simulink model "c00003M_harness"  (R2018a)
settings: Solver=ode3  StartTime=0.0  StopTime=10.0  RelTol=1e-3  EnableMultiTasking=on
undefined symbols (not defined in the file): b, DiscIntNeverNeededParam, J, K, L, PosMinimaW3, PosMinimaW4, R, sigbuilder_block
(part 59 of 73)

== stateflow chart c00003M_harness/M023/Cyber/WL1/Chart1 ==
  state Bajand_hasta_abajo
    entry: W = -1;
  state Bajando
    entry: W = -1;
  state Idle
    entry:W = 0;
  state Subiendo_hasta_arriba
    entry: W = 1;
  state Subiendo
    entry: W = 1;
  Subiendo -> Bajand_hasta_abajo [order 4] : [UI==4]
  Bajand_hasta_abajo -> Bajando [order 2] : [UI==3]
  Subiendo -> Bajando [order 3] : [UI==3]
  Bajando -> Bajand_hasta_abajo [order 2] : [UI==4]
  Idle -> Bajando [order 3] : [UI==3&&S>0]
  Subiendo_hasta_arriba -> Bajand_hasta_abajo [order 3] : [UI==4]
  Idle -> Bajand_hasta_abajo [order 4] : [UI==4&&S>0]
  Bajando -> Subiendo [order 3] : [UI==1]
  Subiendo_hasta_arriba -> Bajando [order 4] : [UI==3]
  Bajand_hasta_abajo -> Subiendo [order 4] : [UI==1]
  Bajand_hasta_abajo -> Idle [order 1] : [S<=0]
  Bajand_hasta_abajo -> Subiendo_hasta_arriba [order 3] : [UI==2]
  Bajando -> Idle [order 1] : [S<=0||UI==0]
  Bajando -> Subiendo_hasta_arriba [order 4] : [UI==2]
  (default) -> Idle
  Idle -> Subiendo_hasta_arriba [order 2] : [UI==2&&S<5]
  Idle -> Subiendo [order 1] : [UI == 1&&S<5]
  Subiendo -> Idle [order 1] : [S>=5||UI==0]
  Subiendo_hasta_arriba -> Idle [order 1] : [S >=5]
  Subiendo_hasta_arriba -> Subiendo [order 2] : [UI ==1]
  Subiendo -> Subiendo_hasta_arriba [order 2] : [UI==2]
  data: S input; UI input; W output double

== stateflow chart c00003M_harness/M023/Cyber/WL2/Chart1 ==
  state Bajand_hasta_abajo
    entry: W = -1;
  state Bajando
    entry: W = -1;
  state Idle
    entry:W = 0;
  state Subiendo_hasta_arriba
    entry: W = 1;
  state Subiendo
    entry: W = 1;
  Subiendo -> Bajand_hasta_abajo [order 4] : [UI==4]
  Bajand_hasta_abajo -> Bajando [order 2] : [UI==3]
  Subiendo -> Bajando [order 3] : [UI==3]
  Bajando -> Bajand_hasta_abajo [order 2] : [UI==4]
  Idle -> Bajando [order 3] : [UI==3&&S>PosMinW3]
  Subiendo_hasta_arriba -> Bajand_hasta_abajo [order 3] : [UI==4]
  Idle -> Bajand_hasta_abajo [order 4] : [UI==4&&S>PosMinW3]
  Bajando -> Subiendo [order 3] : [UI==1]
  Subiendo_hasta_arriba -> Bajando [order 4] : [UI==3]
  Bajand_hasta_abajo -> Subiendo [order 4] : [UI==1]
  Bajand_hasta_abajo -> Idle [order 1] : [S<=PosMinW3]
  Bajand_hasta_abajo -> Subiendo_hasta_arriba [order 3] : [UI==2]
  Bajando -> Idle [order 1] : [S<=PosMinW3||UI==0]
  Bajando -> Subiendo_hasta_arriba [order 4] : [UI==2]
  (default) -> Idle
  Idle -> Subiendo_hasta_arriba [order 2] : [UI==2&&S<5]
  Idle -> Subiendo [order 1] : [UI == 1&&S<5]
  Subiendo -> Idle [order 1] : [S>=5||UI==0]
  Subiendo_hasta_arriba -> Idle [order 1] : [S >=5]
  Subiendo_hasta_arriba -> Subiendo [order 2] : [UI ==1]
  Subiendo -> Subiendo_hasta_arriba [order 2] : [UI==2]
  data: S input; UI input; W output double; PosMinW3 input

== stateflow chart c00003M_harness/M023/Cyber/WL3/Chart2 ==
  state Bajand_hasta_abajo
    entry: W = -1;
  state Bajando
    entry: W = -1;
  state Idle
    entry:W = 0;
  state Subiendo_hasta_arriba
    entry: W = 1;
  state Subiendo
    entry: W = 1;
  Subiendo -> Bajand_hasta_abajo [order 4] : [UI==4]
  Bajand_hasta_abajo -> Bajando [order 2] : [UI==3]
  Subiendo -> Bajando [order 3] : [UI==3]
  Bajando -> Bajand_hasta_abajo [order 2] : [UI==4]
  Idle -> Bajando [order 3] : [UI==3&&S>PosMinW4]
  Subiendo_hasta_arriba -> Bajand_hasta_abajo [order 3] : [UI==4]
  Idle -> Bajand_hasta_abajo [order 4] : [UI==4&&S>PosMinW4]
  Bajando -> Subiendo [order 3] : [UI==1]
  Subiendo_hasta_arriba -> Bajando [order 4] : [UI==3]
  Bajand_hasta_abajo -> Subiendo [order 4] : [UI==1]
  Bajand_hasta_abajo -> Idle [order 1] : [S<=PosMinW4]
  Bajand_hasta_abajo -> Subiendo_hasta_arriba [order 3] : [UI==2]
  Bajando -> Idle [order 1] : [S<=PosMinW4||UI==0]
  Bajando -> Subiendo_hasta_arriba [order 4] : [UI==2]
  (default) -> Idle
  Idle -> Subiendo_hasta_arriba [order 2] : [UI==2&&S<5]
  Idle -> Subiendo [order 1] : [UI == 1&&S<5]
  Subiendo -> Idle [order 1] : [S>=5||UI==0]
  Subiendo_hasta_arriba -> Idle [order 1] : [S >=5]
  Subiendo_hasta_arriba -> Subiendo [order 2] : [UI ==1]
  Subiendo -> Subiendo_hasta_arriba [order 2] : [UI==2]
  data: S input; UI input; W output double; PosMinW4 input

== stateflow chart c00003M_harness/M024/Cyber/WL/Chart ==
  state Bajand_hasta_abajo
    entry: W = -1;
  state Bajando
    entry: W = -1;
  state Idle
    entry:W = 0;
  state Subiendo_hasta_arriba
    entry: W = 1;
  state Subiendo
    entry: W = 1;
  Subiendo -> Bajand_hasta_abajo [order 4] : [UI==4]
  Bajand_hasta_abajo -> Bajando [order 2] : [UI==3]
  Subiendo -> Bajando [order 3] : [UI==3]
  Bajando -> Bajand_hasta_abajo [order 2] : [UI==4]
  Idle -> Bajando [order 3] : [UI==3&&S>0]
  Subiendo_hasta_arriba -> Bajand_hasta_abajo [order 3] : [UI==4]
  Idle -> Bajand_hasta_abajo [order 4] : [UI==4&&S>0]
  Bajando -> Subiendo [order 3] : [UI==1]
  Subiendo_hasta_arriba -> Bajando [order 4] : [UI==3]
  Bajand_hasta_abajo -> Subiendo [order 4] : [UI==1]
  Bajand_hasta_abajo -> Idle [order 1] : [S<=0]
  Bajand_hasta_abajo -> Subiendo_hasta_arriba [order 3] : [UI==2]
  Bajando -> Idle [order 1] : [S<=0||UI==0]
  Bajando -> Subiendo_hasta_arriba [order 4] : [UI==2]
  (default) -> Idle
  Idle -> Subiendo_hasta_arriba [order 2] : [UI==2&&S<5]
  Idle -> Subiendo [order 1] : [UI == 1&&S<5]
  Subiendo -> Idle [order 1] : [S>=5||UI==0]
  Subiendo_hasta_arriba -> Idle [order 1] : [S >=5]
  Subiendo_hasta_arriba -> Subiendo [order 2] : [UI ==1]
  Subiendo -> Subiendo_hasta_arriba [order 2] : [UI==2]
  data: S input; UI input; W output double

== stateflow chart c00003M_harness/M024/Cyber/WL1/Chart1 ==
  state Bajand_hasta_abajo
    entry: W = -1;
  state Bajando
    entry: W = -1;
  state Idle
    entry:W = 1;
  state Subiendo_hasta_arriba
    entry: W = 1;
  state Subiendo
    entry: W = 1;
  Subiendo -> Bajand_hasta_abajo [order 4] : [UI==4]
  Bajand_hasta_abajo -> Bajando [order 2] : [UI==3]
  Subiendo -> Bajando [order 3] : [UI==3]
  Bajando -> Bajand_hasta_abajo [order 2] : [UI==4]
  Idle -> Bajando [order 3] : [UI==3&&S>0]
  Subiendo_hasta_arriba -> Bajand_hasta_abajo [order 3] : [UI==4]
  Idle -> Bajand_hasta_abajo [order 4] : [UI==4&&S>0]
  Bajando -> Subiendo [order 3] : [UI==1]
  Subiendo_hasta_arriba -> Bajando [order 4] : [UI==3]
  Bajand_hasta_abajo -> Subiendo [order 4] : [UI==1]
  Bajand_hasta_abajo -> Idle [order 1] : [S<=0]
  Bajand_hasta_abajo -> Subiendo_hasta_arriba [order 3] : [UI==2]
  Bajando -> Idle [order 1] : [S<=0||UI==0]
  Bajando -> Subiendo_hasta_arriba [order 4] : [UI==2]
  (default) -> Idle
  Idle -> Subiendo_hasta_arriba [order 2] : [UI==2&&S<5]
  Idle -> Subiendo [order 1] : [UI == 1&&S<5]
  Subiendo -> Idle [order 1] : [S>=5||UI==0]
  Subiendo_hasta_arriba -> Idle [order 1] : [S >=5]
  Subiendo_hasta_arriba -> Subiendo [order 2] : [UI ==1]
  Subiendo -> Subiendo_hasta_arriba [order 2] : [UI==2]
  data: S input; UI input; W output double

== stateflow chart c00003M_harness/M024/Cyber/WL2/Chart1 ==
  state Bajand_hasta_abajo
    entry: W = -1;
  state Bajando
    entry: W = -1;
  state Idle
    entry:W = 0;
  state Subiendo_hasta_arriba
    entry: W = 1;
  state Subiendo
    entry: W = 1;
  Subiendo -> Bajand_hasta_abajo [order 4] : [UI==4]
  Bajand_hasta_abajo -> Bajando [order 2] : [UI==3]
  Subiendo -> Bajando [order 3] : [UI==3]
  Bajando -> Bajand_hasta_abajo [order 2] : [UI==4]
  Idle -> Bajando [order 3] : [UI==3&&S>PosMinW3]
  Subiendo_hasta_arriba -> Bajand_hasta_abajo [order 3] : [UI==4]
  Idle -> Bajand_hasta_abajo [order 4] : [UI==4&&S>PosMinW3]
  Bajando -> Subiendo [order 3] : [UI==1]
  Subiendo_hasta_arriba -> Bajando [order 4] : [UI==3]
  Bajand_hasta_abajo -> Subiendo [order 4] : [UI==1]
  Bajand_hasta_abajo -> Idle [order 1] : [S<=PosMinW3]
  Bajand_hasta_abajo -> Subiendo_hasta_arriba [order 3] : [UI==2]
  Bajando -> Idle [order 1] : [S<=PosMinW3||UI==0]
  Bajando -> Subiendo_hasta_arriba [order 4] : [UI==2]
  (default) -> Idle
  Idle -> Subiendo_hasta_arriba [order 2] : [UI==2&&S<5]
  Idle -> Subiendo [order 1] : [UI == 1&&S<5]
  Subiendo -> Idle [order 1] : [S>=5||UI==0]
  Subiendo_hasta_arriba -> Idle [order 1] : [S >=5]
  Subiendo_hasta_arriba -> Subiendo [order 2] : [UI ==1]
  Subiendo -> Subiendo_hasta_arriba [order 2] : [UI==2]
  data: S input; UI input; W output double; PosMinW3 input

== stateflow chart c00003M_harness/M024/Cyber/WL3/Chart2 ==
  state Bajand_hasta_abajo
    entry: W = -1;
  state Bajando
    entry: W = -1;
  state Idle
    entry:W = 0;
  state Subiendo_hasta_arriba
    entry: W = 1;
  state Subiendo
    entry: W = 1;
  Subiendo -> Bajand_hasta_abajo [order 4] : [UI==4]
  Bajand_hasta_abajo -> Bajando [order 2] : [UI==3]
  Subiendo -> Bajando [order 3] : [UI==3]
  Bajando -> Bajand_hasta_abajo [order 2] : [UI==4]
  Idle -> Bajando [order 3] : [UI==3&&S>PosMinW4]
  Subiendo_hasta_arriba -> Bajand_hasta_abajo [order 3] : [UI==4]
  Idle -> Bajand_hasta_abajo [order 4] : [UI==4&&S>PosMinW4]
  Bajando -> Subiendo [order 3] : [UI==1]
  Subiendo_hasta_arriba -> Bajando [order 4] : [UI==3]
  Bajand_hasta_abajo -> Subiendo [order 4] : [UI==1]
  Bajand_hasta_abajo -> Idle [order 1] : [S<=PosMinW4]
  Bajand_hasta_abajo -> Subiendo_hasta_arriba [order 3] : [UI==2]
  Bajando -> Idle [order 1] : [S<=PosMinW4||UI==0]
  Bajando -> Subiendo_hasta_arriba [order 4] : [UI==2]
  (default) -> Idle
  Idle -> Subiendo_hasta_arriba [order 2] : [UI==2&&S<5]
  Idle -> Subiendo [order 1] : [UI == 1&&S<5]
  Subiendo -> Idle [order 1] : [S>=5||UI==0]
  Subiendo_hasta_arriba -> Idle [order 1] : [S >=5]
  Subiendo_hasta_arriba -> Subiendo [order 2] : [UI ==1]
  Subiendo -> Subiendo_hasta_arriba [order 2] : [UI==2]
  data: S input; UI input; W output double; PosMinW4 input

== stateflow chart c00003M_harness/M025/Cyber/WL/Chart ==
  state Bajand_hasta_abajo
    entry: W = -1;
  state Bajando
    entry: W = -1;
  state Idle
    entry:W = 0;
  state Subiendo_hasta_arriba
    entry: W = 1;
  state Subiendo
    entry: W = 1;
  Subiendo -> Bajand_hasta_abajo [order 4] : [UI==4]
  Bajand_hasta_abajo -> Bajando [order 2] : [UI==3]
  Subiendo -> Bajando [order 3] : [UI==3]
  Bajando -> Bajand_hasta_abajo [order 2] : [UI==4]
  Idle -> Bajando [order 3] : [UI==3&&S>0]
  Subiendo_hasta_arriba -> Bajand_hasta_abajo [order 3] : [UI==4]
  Idle -> Bajand_hasta_abajo [order 4] : [UI==4&&S>0]
  Bajando -> Subiendo [order 3] : [UI==1]
  Subiendo_hasta_arriba -> Bajando [order 4] : [UI==3]
  Bajand_hasta_abajo -> Subiendo [order 4] : [UI==1]
  Bajand_hasta_abajo -> Idle [order 1] : [S<=0]
  Bajand_hasta_abajo -> Subiendo_hasta_arriba [order 3] : [UI==2]
  Bajando -> Idle [order 1] : [S<=0||UI==0]
  Bajando -> Subiendo_hasta_arriba [order 4] : [UI==2]
  (default) -> Idle
  Idle -> Subiendo_hasta_arriba [order 2] : [UI==2&&S<5]
  Idle -> Subiendo [order 1] : [UI == 1&&S<5]
  Subiendo -> Idle [order 1] : [S>=5||UI==0]
  Subiendo_hasta_arriba -> Idle [order 1] : [S >=5]
  Subiendo_hasta_arriba -> Subiendo [order 2] : [UI ==1]
  Subiendo -> Subiendo_hasta_arriba [order 2] : [UI==2]
  data: S input; UI input; W output double

== stateflow chart c00003M_harness/M025/Cyber/WL1/Chart1 ==
  state Bajand_hasta_abajo
    entry: W = -1;
  state Bajando
    entry: W = -1;
  state Idle
    entry:W = 0;
  state Subiendo_hasta_arriba
    entry: W = 1;
  state Subiendo
    entry: W = 1;
  Subiendo -> Bajand_hasta_abajo [order 4] : [UI==4]
  Bajand_hasta_abajo -> Bajando [order 2] : [UI==3]
  Subiendo -> Bajando [order 3] : [UI==3]
  Bajando -> Bajand_hasta_abajo [order 2] : [UI==4]
  Idle -> Bajando [order 3] : [UI==3&&S>0]
  Subiendo_hasta_arriba -> Bajand_hasta_abajo [order 3] : [UI==4]
  Idle -> Bajand_hasta_abajo [order 4] : [UI==4&&S>0]
  Bajando -> Subiendo [order 3] : [UI==1]
  Subiendo_hasta_arriba -> Bajando [order 4] : [UI==3]
  Bajand_hasta_abajo -> Subiendo [order 4] : [UI==1]
  Bajand_hasta_abajo -> Idle [order 1] : [S<=0]
  Bajand_hasta_abajo -> Subiendo_hasta_arriba [order 3] : [UI==2]
  Bajando -> Idle [order 1] : [S<=0||UI==0]
  Bajando -> Subiendo_hasta_arriba [order 4] : [UI==2]
  (default) -> Idle
  Idle -> Subiendo_hasta_arriba [order 2] : [UI==2&&S<5]
  Idle -> Subiendo [order 1] : [UI == 1&&S<5]
  Subiendo -> Idle [order 1] : [S>=5||UI==0]
  Subiendo_hasta_arriba -> Idle [order 1] : [S >=5]
  Subiendo_hasta_arriba -> Subiendo [order 2] : [UI ==1]
  Subiendo -> Subiendo_hasta_arriba [order 2] : [UI==2]
  data: S input; UI input; W output double

== stateflow chart c00003M_harness/M025/Cyber/WL2/Chart1 ==
  state Bajand_hasta_abajo
    entry: W = -1;
  state Bajando
    entry: W = -1;
  state Idle
    entry:W = 1;
  state Subiendo_hasta_arriba
    entry: W = 1;
  state Subiendo
    entry: W = 1;
  Subiendo -> Bajand_hasta_abajo [order 4] : [UI==4]
  Bajand_hasta_abajo -> Bajando [order 2] : [UI==3]
  Subiendo -> Bajando [order 3] : [UI==3]
  Bajando -> Bajand_hasta_abajo [order 2] : [UI==4]
  Idle -> Bajando [order 3] : [UI==3&&S>PosMinW3]
  Subiendo_hasta_arriba -> Bajand_hasta_abajo [order 3] : [UI==4]
  Idle -> Bajand_hasta_abajo [order 4] : [UI==4&&S>PosMinW3]
  Bajando -> Subiendo [order 3] : [UI==1]
  Subiendo_hasta_arriba -> Bajando [order 4] : [UI==3]
  Bajand_hasta_abajo -> Subiendo [order 4] : [UI==1]
  Bajand_hasta_abajo -> Idle [order 1] : [S<=PosMinW3]
  Bajand_hasta_abajo -> Subiendo_hasta_arriba [order 3] : [UI==2]
  Bajando -> Idle [order 1] : [S<=PosMinW3||UI==0]
  Bajando -> Subiendo_hasta_arriba [order 4] : [UI==2]
  (default) -> Idle
  Idle -> Subiendo_hasta_arriba [order 2] : [UI==2&&S<5]
  Idle -> Subiendo [order 1] : [UI == 1&&S<5]
  Subiendo -> Idle [order 1] : [S>=5||UI==0]
  Subiendo_hasta_arriba -> Idle [order 1] : [S >=5]
  Subiendo_hasta_arriba -> Subiendo [order 2] : [UI ==1]
  Subiendo -> Subiendo_hasta_arriba [order 2] : [UI==2]
  data: S input; UI input; W output double; PosMinW3 input

== stateflow chart c00003M_harness/M025/Cyber/WL3/Chart2 ==
  state Bajand_hasta_abajo
    entry: W = -1;
  state Bajando
    entry: W = -1;
  state Idle
    entry:W = 0;
  state Subiendo_hasta_arriba
    entry: W = 1;
  state Subiendo
    entry: W = 1;
  Subiendo -> Bajand_hasta_abajo [order 4] : [UI==4]
  Bajand_hasta_abajo -> Bajando [order 2] : [UI==3]
  Subiendo -> Bajando [order 3] : [UI==3]
  Bajando -> Bajand_hasta_abajo [order 2] : [UI==4]
  Idle -> Bajando [order 3] : [UI==3&&S>PosMinW4]
  Subiendo_hasta_arriba -> Bajand_hasta_abajo [order 3] : [UI==4]
  Idle -> Bajand_hasta_abajo [order 4] : [UI==4&&S>PosMinW4]
  Bajando -> Subiendo [order 3] : [UI==1]
  Subiendo_hasta_arriba -> Bajando [order 4] : [UI==3]
  Bajand_hasta_abajo -> Subiendo [order 4] : [UI==1]
  Bajand_hasta_abajo -> Idle [order 1] : [S<=PosMinW4]
  Bajand_hasta_abajo -> Subiendo_hasta_arriba [order 3] : [UI==2]
  Bajando -> Idle [order 1] : [S<=PosMinW4||UI==0]
  Bajando -> Subiendo_hasta_arriba [order 4] : [UI==2]
  (default) -> Idle
  Idle -> Subiendo_hasta_arriba [order 2] : [UI==2&&S<5]
  Idle -> Subiendo [order 1] : [UI == 1&&S<5]
  Subiendo -> Idle [order 1] : [S>=5||UI==0]
  Subiendo_hasta_arriba -> Idle [order 1] : [S >=5]
  Subiendo_hasta_arriba -> Subiendo [order 2] : [UI ==1]
  Subiendo -> Subiendo_hasta_arriba [order 2] : [UI==2]
  data: S input; UI input; W output double; PosMinW4 input

== stateflow chart c00003M_harness/M026/Cyber/WL/Chart ==
  state Bajand_hasta_abajo
    entry: W = -1;
  state Bajando
    entry: W = -1;
  state Idle
    entry:W = 0;
  state Subiendo_hasta_arriba
    entry: W = 1;
  state Subiendo
    entry: W = 1;
  Subiendo -> Bajand_hasta_abajo [order 4] : [UI==4]
  Bajand_hasta_abajo -> Bajando [order 2] : [UI==3]
  Subiendo -> Bajando [order 3] : [UI==3]
  Bajando -> Bajand_hasta_abajo [order 2] : [UI==4]
  Idle -> Bajando [order 3] : [UI==3&&S>0]
  Subiendo_hasta_arriba -> Bajand_hasta_abajo [order 3] : [UI==4]
  Idle -> Bajand_hasta_abajo [order 4] : [UI==4&&S>0]
  Bajando -> Subiendo [order 3] : [UI==1]
  Subiendo_hasta_arriba -> Bajando [order 4] : [UI==3]
  Bajand_hasta_abajo -> Subiendo [order 4] : [UI==1]
  Bajand_hasta_abajo -> Idle [order 1] : [S<=0]
  Bajand_hasta_abajo -> Subiendo_hasta_arriba [order 3] : [UI==2]
  Bajando -> Idle [order 1] : [S<=0||UI==0]
  Bajando -> Subiendo_hasta_arriba [order 4] : [UI==2]
  (default) -> Idle
  Idle -> Subiendo_hasta_arriba [order 2] : [UI==2&&S<5]
  Idle -> Subiendo [order 1] : [UI == 1&&S<5]
  Subiendo -> Idle [order 1] : [S>=5||UI==0]
  Subiendo_hasta_arriba -> Idle [order 1] : [S >=5]
  Subiendo_hasta_arriba -> Subiendo [order 2] : [UI ==1]
  Subiendo -> Subiendo_hasta_arriba [order 2] : [UI==2]
  data: S input; UI input; W output double

== stateflow chart c00003M_harness/M026/Cyber/WL1/Chart1 ==
  state Bajand_hasta_abajo
    entry: W = -1;
  state Bajando
    entry: W = -1;
  state Idle
    entry:W = 0;
  state Subiendo_hasta_arriba
    entry: W = 1;
  state Subiendo
    entry: W = 1;
  Subiendo -> Bajand_hasta_abajo [order 4] : [UI==4]
  Bajand_hasta_abajo -> Bajando [order 2] : [UI==3]
  Subiendo -> Bajando [order 3] : [UI==3]
  Bajando -> Bajand_hasta_abajo [order 2] : [UI==4]
  Idle -> Bajando [order 3] : [UI==3&&S>0]
  Subiendo_hasta_arriba -> Bajand_hasta_abajo [order 3] : [UI==4]
  Idle -> Bajand_hasta_abajo [order 4] : [UI==4&&S>0]
  Bajando -> Subiendo [order 3] : [UI==1]
  Subiendo_hasta_arriba -> Bajando [order 4] : [UI==3]
  Bajand_hasta_abajo -> Subiendo [order 4] : [UI==1]
  Bajand_hasta_abajo -> Idle [order 1] : [S<=0]
  Bajand_hasta_abajo -> Subiendo_hasta_arriba [order 3] : [UI==2]
  Bajando -> Idle [order 1] : [S<=0||UI==0]
  Bajando -> Subiendo_hasta_arriba [order 4] : [UI==2]
  (default) -> Idle
  Idle -> Subiendo_hasta_arriba [order 2] : [UI==2&&S<5]
  Idle -> Subiendo [order 1] : [UI == 1&&S<5]
  Subiendo -> Idle [order 1] : [S>=5||UI==0]
  Subiendo_hasta_arriba -> Idle [order 1] : [S >=5]
  Subiendo_hasta_arriba -> Subiendo [order 2] : [UI ==1]
  Subiendo -> Subiendo_hasta_arriba [order 2] : [UI==2]
  data: S input; UI input; W output double

== stateflow chart c00003M_harness/M026/Cyber/WL2/Chart1 ==
  state Bajand_hasta_abajo
    entry: W = -1;
  state Bajando
    entry: W = -1;
  state Idle
    entry:W = 0;
  state Subiendo_hasta_arriba
    entry: W = 1;
  state Subiendo
    entry: W = 1;
  Subiendo -> Bajand_hasta_abajo [order 4] : [UI==4]
  Bajand_hasta_abajo -> Bajando [order 2] : [UI==3]
  Subiendo -> Bajando [order 3] : [UI==3]
  Bajando -> Bajand_hasta_abajo [order 2] : [UI==4]
  Idle -> Bajando [order 3] : [UI==3&&S>PosMinW3]
  Subiendo_hasta_arriba -> Bajand_hasta_abajo [order 3] : [UI==4]
  Idle -> Bajand_hasta_abajo [order 4] : [UI==4&&S>PosMinW3]
  Bajando -> Subiendo [order 3] : [UI==1]
  Subiendo_hasta_arriba -> Bajando [order 4] : [UI==3]
  Bajand_hasta_abajo -> Subiendo [order 4] : [UI==1]
  Bajand_hasta_abajo -> Idle [order 1] : [S<=PosMinW3]
  Bajand_hasta_abajo -> Subiendo_hasta_arriba [order 3] : [UI==2]
  Bajando -> Idle [order 1] : [S<=PosMinW3||UI==0]
  Bajando -> Subiendo_hasta_arriba [order 4] : [UI==2]
  (default) -> Idle
  Idle -> Subiendo_hasta_arriba [order 2] : [UI==2&&S<5]
  Idle -> Subiendo [order 1] : [UI == 1&&S<5]
  Subiendo -> Idle [order 1] : [S>=5||UI==0]
  Subiendo_hasta_arriba -> Idle [order 1] : [S >=5]
  Subiendo_hasta_arriba -> Subiendo [order 2] : [UI ==1]
  Subiendo -> Subiendo_hasta_arriba [order 2] : [UI==2]
  data: S input; UI input; W output double; PosMinW3 input

== stateflow chart c00003M_harness/M026/Cyber/WL3/Chart2 ==
  state Bajand_hasta_abajo
    entry: W = -1;
  state Bajando
    entry: W = -1;
  state Idle
    entry:W = 1;
  state Subiendo_hasta_arriba
    entry: W = 1;
  state Subiendo
    entry: W = 1;
  Subiendo -> Bajand_hasta_abajo [order 4] : [UI==4]
  Bajand_hasta_abajo -> Bajando [order 2] : [UI==3]
  Subiendo -> Bajando [order 3] : [UI==3]
  Bajando -> Bajand_hasta_abajo [order 2] : [UI==4]
  Idle -> Bajando [order 3] : [UI==3&&S>PosMinW4]
  Subiendo_hasta_arriba -> Bajand_hasta_abajo [order 3] : [UI==4]
  Idle -> Bajand_hasta_abajo [order 4] : [UI==4&&S>PosMinW4]
  Bajando -> Subiendo [order 3] : [UI==1]
  Subiendo_hasta_arriba -> Bajando [order 4] : [UI==3]
  Bajand_hasta_abajo -> Subiendo [order 4] : [UI==1]
  Bajand_hasta_abajo -> Idle [order 1] : [S<=PosMinW4]
  Bajand_hasta_abajo -> Subiendo_hasta_arriba [order 3] : [UI==2]
  Bajando -> Idle [order 1] : [S<=PosMinW4||UI==0]
  Bajando -> Subiendo_hasta_arriba [order 4] : [UI==2]
  (default) -> Idle
  Idle -> Subiendo_hasta_arriba [order 2] : [UI==2&&S<5]
  Idle -> Subiendo [order 1] : [UI == 1&&S<5]
  Subiendo -> Idle [order 1] : [S>=5||UI==0]
  Subiendo_hasta_arriba -> Idle [order 1] : [S >=5]
  Subiendo_hasta_arriba -> Subiendo [order 2] : [UI ==1]
  Subiendo -> Subiendo_hasta_arriba [order 2] : [UI==2]
  data: S input; UI input; W output double; PosMinW4 input

== stateflow chart c00003M_harness/M027/Cyber/WL/Chart ==
  state Bajand_hasta_abajo
    entry: W = -1;
  state Bajando
    entry: W = -1;
  state Idle
    entry:W = 0;
  state Subiendo_hasta_arriba
    entry: W = 1;
  state Subiendo
    entry: W = 0;
  Subiendo -> Bajand_hasta_abajo [order 4] : [UI==4]
  Bajand_hasta_abajo -> Bajando [order 2] : [UI==3]
  Subiendo -> Bajando [order 3] : [UI==3]
  Bajando -> Bajand_hasta_abajo [order 2] : [UI==4]
  Idle -> Bajando [order 3] : [UI==3&&S>0]
  Subiendo_hasta_arriba -> Bajand_hasta_abajo [order 3] : [UI==4]
  Idle -> Bajand_hasta_abajo [order 4] : [UI==4&&S>0]
  Bajando -> Subiendo [order 3] : [UI==1]
  Subiendo_hasta_arriba -> Bajando [order 4] : [UI==3]
  Bajand_hasta_abajo -> Subiendo [order 4] : [UI==1]
  Bajand_hasta_abajo -> Idle [order 1] : [S<=0]
  Bajand_hasta_abajo -> Subiendo_hasta_arriba [order 3] : [UI==2]
  Bajando -> Idle [order 1] : [S<=0||UI==0]
  Bajando -> Subiendo_hasta_arriba [order 4] : [UI==2]
  (default) -> Idle
  Idle -> Subiendo_hasta_arriba [order 2] : [UI==2&&S<5]
  Idle -> Subiendo [order 1] : [UI == 1&&S<5]
  Subiendo -> Idle [order 1] : [S>=5||UI==0]
  Subiendo_hasta_arriba -> Idle [order 1] : [S >=5]
  Subiendo_hasta_arriba -> Subiendo [order 2] : [UI ==1]
  Subiendo -> Subiendo_hasta_arriba [order 2] : [UI==2]
  data: S input; UI input; W output double

== stateflow chart c00003M_harness/M027/Cyber/WL1/Chart1 ==
  state Bajand_hasta_abajo
    entry: W = -1;
  state Bajando
    entry: W = -1;
  state Idle
    entry:W = 0;
  state Subiendo_hasta_arriba
    entry: W = 1;
  state Subiendo
    entry: W = 1;
  Subiendo -> Bajand_hasta_abajo [order 4] : [UI==4]
  Bajand_hasta_abajo -> Bajando [order 2] : [UI==3]
  Subiendo -> Bajando [order 3] : [UI==3]
  Bajando -> Bajand_hasta_abajo [order 2] : [UI==4]
  Idle -> Bajando [order 3] : [UI==3&&S>0]
  Subiendo_hasta_arriba -> Bajand_hasta_abajo [order 3] : [UI==4]
  Idle -> Bajand_hasta_abajo [order 4] : [UI==4&&S>0]
  Bajando -> Subiendo [order 3] : [UI==1]
  Subiendo_hasta_arriba -> Bajando [order 4] : [UI==3]
  Bajand_hasta_abajo -> Subiendo [order 4] : [UI==1]
  Bajand_hasta_abajo -> Idle [order 1] : [S<=0]
  Bajand_hasta_abajo -> Subiendo_hasta_arriba [order 3] : [UI==2]
  Bajando -> Idle [order 1] : [S<=0||UI==0]
  Bajando -> Subiendo_hasta_arriba [order 4] : [UI==2]
  (default) -> Idle
  Idle -> Subiendo_hasta_arriba [order 2] : [UI==2&&S<5]
  Idle -> Subiendo [order 1] : [UI == 1&&S<5]
  Subiendo -> Idle [order 1] : [S>=5||UI==0]
  Subiendo_hasta_arriba -> Idle [order 1] : [S >=5]
  Subiendo_hasta_arriba -> Subiendo [order 2] : [UI ==1]
  Subiendo -> Subiendo_hasta_arriba [order 2] : [UI==2]
  data: S input; UI input; W output double

== stateflow chart c00003M_harness/M027/Cyber/WL2/Chart1 ==
  state Bajand_hasta_abajo
    entry: W = -1;
  state Bajando
    entry: W = -1;
  state Idle
    entry:W = 0;
  state Subiendo_hasta_arriba
    entry: W = 1;
  state Subiendo
    entry: W = 1;
  Subiendo -> Bajand_hasta_abajo [order 4] : [UI==4]
  Bajand_hasta_abajo -> Bajando [order 2] : [UI==3]
  Subiendo -> Bajando [order 3] : [UI==3]
  Bajando -> Bajand_hasta_abajo [order 2] : [UI==4]
  Idle -> Bajando [order 3] : [UI==3&&S>PosMinW3]
  Subiendo_hasta_arriba -> Bajand_hasta_abajo [order 3] : [UI==4]
  Idle -> Bajand_hasta_abajo [order 4] : [UI==4&&S>PosMinW3]
  Bajando -> Subiendo [order 3] : [UI==1]
  Subiendo_hasta_arriba -> Bajando [order 4] : [UI==3]
  Bajand_hasta_abajo -> Subiendo [order 4] : [UI==1]
  Bajand_hasta_abajo -> Idle [order 1] : [S<=PosMinW3]
  Bajand_hasta_abajo -> Subiendo_hasta_arriba [order 3] : [UI==2]
  Bajando -> Idle [order 1] : [S<=PosMinW3||UI==0]
  Bajando -> Subiendo_hasta_arriba [order 4] : [UI==2]
  (default) -> Idle
  Idle -> Subiendo_hasta_arriba [order 2] : [UI==2&&S<5]
  Idle -> Subiendo [order 1] : [UI == 1&&S<5]
  Subiendo -> Idle [order 1] : [S>=5||UI==0]
  Subiendo_hasta_arriba -> Idle [order 1] : [S >=5]
  Subiendo_hasta_arriba -> Subiendo [order 2] : [UI ==1]
  Subiendo -> Subiendo_hasta_arriba [order 2] : [UI==2]
  data: S input; UI input; W output double; PosMinW3 input

== stateflow chart c00003M_harness/M027/Cyber/WL3/Chart2 ==
  state Bajand_hasta_abajo
    entry: W = -1;
  state Bajando
    entry: W = -1;
  state Idle
    entry:W = 0;
  state Subiendo_hasta_arriba
    entry: W = 1;
  state Subiendo
    entry: W = 1;
  Subiendo -> Bajand_hasta_abajo [order 4] : [UI==4]
  Bajand_hasta_abajo -> Bajando [order 2] : [UI==3]
  Subiendo -> Bajando [order 3] : [UI==3]
  Bajando -> Bajand_hasta_abajo [order 2] : [UI==4]
  Idle -> Bajando [order 3] : [UI==3&&S>PosMinW4]
  Subiendo_hasta_arriba -> Bajand_hasta_abajo [order 3] : [UI==4]
  Idle -> Bajand_hasta_abajo [order 4] : [UI==4&&S>PosMinW4]
  Bajando -> Subiendo [order 3] : [UI==1]
  Subiendo_hasta_arriba -> Bajando [order 4] : [UI==3]
  Bajand_hasta_abajo -> Subiendo [order 4] : [UI==1]
  Bajand_hasta_abajo -> Idle [order 1] : [S<=PosMinW4]
  Bajand_hasta_abajo -> Subiendo_hasta_arriba [order 3] : [UI==2]
  Bajando -> Idle [order 1] : [S<=PosMinW4||UI==0]
  Bajando -> Subiendo_hasta_arriba [order 4] : [UI==2]
  (default) -> Idle
  Idle -> Subiendo_hasta_arriba [order 2] : [UI==2&&S<5]
  Idle -> Subiendo [order 1] : [UI == 1&&S<5]
  Subiendo -> Idle [order 1] : [S>=5||UI==0]
  Subiendo_hasta_arriba -> Idle [order 1] : [S >=5]
  Subiendo_hasta_arriba -> Subiendo [order 2] : [UI ==1]
  Subiendo -> Subiendo_hasta_arriba [order 2] : [UI==2]
  data: S input; UI input; W output double; PosMinW4 input

== stateflow chart c00003M_harness/M028/Cyber/WL/Chart ==
  state Bajand_hasta_abajo
    entry: W = -1;
  state Bajando
    entry: W = -1;
  state Idle
    entry:W = 0;
  state Subiendo_hasta_arriba
    entry: W = 1;
  state Subiendo
    entry: W = 1;
  Subiendo -> Bajand_hasta_abajo [order 4] : [UI==4]
  Bajand_hasta_abajo -> Bajando [order 2] : [UI==3]
  Subiendo -> Bajando [order 3] : [UI==3]
  Bajando -> Bajand_hasta_abajo [order 2] : [UI==4]
  Idle -> Bajando [order 3] : [UI==3&&S>0]
  Subiendo_hasta_arriba -> Bajand_hasta_abajo [order 3] : [UI==4]
  Idle -> Bajand_hasta_abajo [order 4] : [UI==4&&S>0]
  Bajando -> Subiendo [order 3] : [UI==1]
  Subiendo_hasta_arriba -> Bajando [order 4] : [UI==3]
  Bajand_hasta_abajo -> Subiendo [order 4] : [UI==1]
  Bajand_hasta_abajo -> Idle [order 1] : [S<=0]
  Bajand_hasta_abajo -> Subiendo_hasta_arriba [order 3] : [UI==2]
  Bajando -> Idle [order 1] : [S<=0||UI==0]
  Bajando -> Subiendo_hasta_arriba [order 4] : [UI==2]
  (default) -> Idle
  Idle -> Subiendo_hasta_arriba [order 2] : [UI==2&&S<5]
  Idle -> Subiendo [order 1] : [UI == 1&&S<5]
  Subiendo -> Idle [order 1] : [S>=5||UI==0]
  Subiendo_hasta_arriba -> Idle [order 1] : [S >=5]
  Subiendo_hasta_arriba -> Subiendo [order 2] : [UI ==1]
  Subiendo -> Subiendo_hasta_arriba [order 2] : [UI==2]
  data: S input; UI input; W output double

== stateflow chart c00003M_harness/M028/Cyber/WL1/Chart1 ==
  state Bajand_hasta_abajo
    entry: W = -1;
  state Bajando
    entry: W = -1;
  state Idle
    entry:W = 0;
  state Subiendo_hasta_arriba
    entry: W = 1;
  state Subiendo
    entry: W = 0;
  Subiendo -> Bajand_hasta_abajo [order 4] : [UI==4]
  Bajand_hasta_abajo -> Bajando [order 2] : [UI==3]
  Subiendo -> Bajando [order 3] : [UI==3]
  Bajando -> Bajand_hasta_abajo [order 2] : [UI==4]
  Idle -> Bajando [order 3] : [UI==3&&S>0]
  Subiendo_hasta_arriba -> Bajand_hasta_abajo [order 3] : [UI==4]
  Idle -> Bajand_hasta_abajo [order 4] : [UI==4&&S>0]
  Bajando -> Subiendo [order 3] : [UI==1]
  Subiendo_hasta_arriba -> Bajando [order 4] : [UI==3]
  Bajand_hasta_abajo -> Subiendo [order 4] : [UI==1]
  Bajand_hasta_abajo -> Idle [order 1] : [S<=0]
  Bajand_hasta_abajo -> Subiendo_hasta_arriba [order 3] : [UI==2]
  Bajando -> Idle [order 1] : [S<=0||UI==0]
  Bajando -> Subiendo_hasta_arriba [order 4] : [UI==2]
  (default) -> Idle
  Idle -> Subiendo_hasta_arriba [order 2] : [UI==2&&S<5]
  Idle -> Subiendo [order 1] : [UI == 1&&S<5]
  Subiendo -> Idle [order 1] : [S>=5||UI==0]
  Subiendo_hasta_arriba -> Idle [order 1] : [S >=5]
  Subiendo_hasta_arriba -> Subiendo [order 2] : [UI ==1]
  Subiendo -> Subiendo_hasta_arriba [order 2] : [UI==2]
  data: S input; UI input; W output double

== stateflow chart c00003M_harness/M028/Cyber/WL2/Chart1 ==
  state Bajand_hasta_abajo
    entry: W = -1;
  state Bajando
    entry: W = -1;
  state Idle
    entry:W = 0;
  state Subiendo_hasta_arriba
    entry: W = 1;
  state Subiendo
    entry: W = 1;
  Subiendo -> Bajand_hasta_abajo [order 4] : [UI==4]
  Bajand_hasta_abajo -> Bajando [order 2] : [UI==3]
  Subiendo -> Bajando [order 3] : [UI==3]
  Bajando -> Bajand_hasta_abajo [order 2] : [UI==4]
  Idle -> Bajando [order 3] : [UI==3&&S>PosMinW3]
  Subiendo_hasta_arriba -> Bajand_hasta_abajo [order 3] : [UI==4]
  Idle -> Bajand_hasta_abajo [order 4] : [UI==4&&S>PosMinW3]
  Bajando -> Subiendo [order 3] : [UI==1]
  Subiendo_hasta_arriba -> Bajando [order 4] : [UI==3]
  Bajand_hasta_abajo -> Subiendo [order 4] : [UI==1]
  Bajand_hasta_abajo -> Idle [order 1] : [S<=PosMinW3]
  Bajand_hasta_abajo -> Subiendo_hasta_arriba [order 3] : [UI==2]
  Bajando -> Idle [order 1] : [S<=PosMinW3||UI==0]
  Bajando -> Subiendo_hasta_arriba [order 4] : [UI==2]
  (default) -> Idle
  Idle -> Subiendo_hasta_arriba [order 2] : [UI==2&&S<5]
  Idle -> Subiendo [order 1] : [UI == 1&&S<5]
  Subiendo -> Idle [order 1] : [S>=5||UI==0]
  Subiendo_hasta_arriba -> Idle [order 1] : [S >=5]
  Subiendo_hasta_arriba -> Subiendo [order 2] : [UI ==1]
  Subiendo -> Subiendo_hasta_arriba [order 2] : [UI==2]
  data: S input; UI input; W output double; PosMinW3 input

== stateflow chart c00003M_harness/M028/Cyber/WL3/Chart2 ==
  state Bajand_hasta_abajo
    entry: W = -1;
  state Bajando
    entry: W = -1;
  state Idle
    entry:W = 0;
  state Subiendo_hasta_arriba
    entry: W = 1;
  state Subiendo
    entry: W = 1;
  Subiendo -> Bajand_hasta_abajo [order 4] : [UI==4]
  Bajand_hasta_abajo -> Bajando [order 2] : [UI==3]
  Subiendo -> Bajando [order 3] : [UI==3]
  Bajando -> Bajand_hasta_abajo [order 2] : [UI==4]
  Idle -> Bajando [order 3] : [UI==3&&S>PosMinW4]
  Subiendo_hasta_arriba -> Bajand_hasta_abajo [order 3] : [UI==4]
  Idle -> Bajand_hasta_abajo [order 4] : [UI==4&&S>PosMinW4]
  Bajando -> Subiendo [order 3] : [UI==1]
  Subiendo_hasta_arriba -> Bajando [order 4] : [UI==3]
  Bajand_hasta_abajo -> Subiendo [order 4] : [UI==1]
  Bajand_hasta_abajo -> Idle [order 1] : [S<=PosMinW4]
  Bajand_hasta_abajo -> Subiendo_hasta_arriba [order 3] : [UI==2]
  Bajando -> Idle [order 1] : [S<=PosMinW4||UI==0]
  Bajando -> Subiendo_hasta_arriba [order 4] : [UI==2]
  (default) -> Idle
  Idle -> Subiendo_hasta_arriba [order 2] : [UI==2&&S<5]
  Idle -> Subiendo [order 1] : [UI == 1&&S<5]
  Subiendo -> Idle [order 1] : [S>=5||UI==0]
  Subiendo_hasta_arriba -> Idle [order 1] : [S >=5]
  Subiendo_hasta_arriba -> Subiendo [order 2] : [UI ==1]
  Subiendo -> Subiendo_hasta_arriba [order 2] : [UI==2]
  data: S input; UI input; W output double; PosMinW4 input

== stateflow chart c00003M_harness/M029/Cyber/WL/Chart ==
  state Bajand_hasta_abajo
    entry: W = -1;
  state Bajando
    entry: W = -1;
  state Idle
    entry:W = 0;
  state Subiendo_hasta_arriba
    entry: W = 1;
  state Subiendo
    entry: W = 1;
  Subiendo -> Bajand_hasta_abajo [order 4] : [UI==4]
  Bajand_hasta_abajo -> Bajando [order 2] : [UI==3]
  Subiendo -> Bajando [order 3] : [UI==3]
  Bajando -> Bajand_hasta_abajo [order 2] : [UI==4]
  Idle -> Bajando [order 3] : [UI==3&&S>0]
  Subiendo_hasta_arriba -> Bajand_hasta_abajo [order 3] : [UI==4]
  Idle -> Bajand_hasta_abajo [order 4] : [UI==4&&S>0]
  Bajando -> Subiendo [order 3] : [UI==1]
  Subiendo_hasta_arriba -> Bajando [order 4] : [UI==3]
  Bajand_hasta_abajo -> Subiendo [order 4] : [UI==1]
  Bajand_hasta_abajo -> Idle [order 1] : [S<=0]
  Bajand_hasta_abajo -> Subiendo_hasta_arriba [order 3] : [UI==2]
  Bajando -> Idle [order 1] : [S<=0||UI==0]
  Bajando -> Subiendo_hasta_arriba [order 4] : [UI==2]
  (default) -> Idle
  Idle -> Subiendo_hasta_arriba [order 2] : [UI==2&&S<5]
  Idle -> Subiendo [order 1] : [UI == 1&&S<5]
  Subiendo -> Idle [order 1] : [S>=5||UI==0]
  Subiendo_hasta_arriba -> Idle [order 1] : [S >=5]
  Subiendo_hasta_arriba -> Subiendo [order 2] : [UI ==1]
  Subiendo -> Subiendo_hasta_arriba [order 2] : [UI==2]
  data: S input; UI input; W output double

== stateflow chart c00003M_harness/M029/Cyber/WL1/Chart1 ==
  state Bajand_hasta_abajo
    entry: W = -1;
  state Bajando
    entry: W = -1;
  state Idle
    entry:W = 0;
  state Subiendo_hasta_arriba
    entry: W = 1;
  state Subiendo
    entry: W = 1;
  Subiendo -> Bajand_hasta_abajo [order 4] : [UI==4]
  Bajand_hasta_abajo -> Bajando [order 2] : [UI==3]
  Subiendo -> Bajando [order 3] : [UI==3]
  Bajando -> Bajand_hasta_abajo [order 2] : [UI==4]
  Idle -> Bajando [order 3] : [UI==3&&S>0]
  Subiendo_hasta_arriba -> Bajand_hasta_abajo [order 3] : [UI==4]
  Idle -> Bajand_hasta_abajo [order 4] : [UI==4&&S>0]
  Bajando -> Subiendo [order 3] : [UI==1]
  Subiendo_hasta_arriba -> Bajando [order 4] : [UI==3]
  Bajand_hasta_abajo -> Subiendo [order 4] : [UI==1]
  Bajand_hasta_abajo -> Idle [order 1] : [S<=0]
  Bajand_hasta_abajo -> Subiendo_hasta_arriba [order 3] : [UI==2]
  Bajando -> Idle [order 1] : [S<=0||UI==0]
  Bajando -> Subiendo_hasta_arriba [order 4] : [UI==2]
  (default) -> Idle
  Idle -> Subiendo_hasta_arriba [order 2] : [UI==2&&S<5]
  Idle -> Subiendo [order 1] : [UI == 1&&S<5]
  Subiendo -> Idle [order 1] : [S>=5||UI==0]
  Subiendo_hasta_arriba -> Idle [order 1] : [S >=5]
  Subiendo_hasta_arriba -> Subiendo [order 2] : [UI ==1]
  Subiendo -> Subiendo_hasta_arriba [order 2] : [UI==2]
  data: S input; UI input; W output double

== stateflow chart c00003M_harness/M029/Cyber/WL2/Chart1 ==
  state Bajand_hasta_abajo
    entry: W = -1;
  state Bajando
    entry: W = -1;
  state Idle
    entry:W = 0;
  state Subiendo_hasta_arriba
    entry: W = 1;
  state Subiendo
    entry: W = 0;
  Subiendo -> Bajand_hasta_abajo [order 4] : [UI==4]
  Bajand_hasta_abajo -> Bajando [order 2] : [UI==3]
  Subiendo -> Bajando [order 3] : [UI==3]
  Bajando -> Bajand_hasta_abajo [order 2] : [UI==4]
  Idle -> Bajando [order 3] : [UI==3&&S>PosMinW3]
  Subiendo_hasta_arriba -> Bajand_hasta_abajo [order 3] : [UI==4]
  Idle -> Bajand_hasta_abajo [order 4] : [UI==4&&S>PosMinW3]
  Bajando -> Subiendo [order 3] : [UI==1]
  Subiendo_hasta_arriba -> Bajando [order 4] : [UI==3]
  Bajand_hasta_abajo -> Subiendo [order 4] : [UI==1]
  Bajand_hasta_abajo -> Idle [order 1] : [S<=PosMinW3]
  Bajand_hasta_abajo -> Subiendo_hasta_arriba [order 3] : [UI==2]
  Bajando -> Idle [order 1] : [S<=PosMinW3||UI==0]
  Bajando -> Subiendo_hasta_arriba [order 4] : [UI==2]
  (default) -> Idle
  Idle -> Subiendo_hasta_arriba [order 2] : [UI==2&&S<5]
  Idle -> Subiendo [order 1] : [UI == 1&&S<5]
  Subiendo -> Idle [order 1] : [S>=5||UI==0]
  Subiendo_hasta_arriba -> Idle [order 1] : [S >=5]
  Subiendo_hasta_arriba -> Subiendo [order 2] : [UI ==1]
  Subiendo -> Subiendo_hasta_arriba [order 2] : [UI==2]
  data: S input; UI input; W output double; PosMinW3 input

== stateflow chart c00003M_harness/M029/Cyber/WL3/Chart2 ==
  state Bajand_hasta_abajo
    entry: W = -1;
  state Bajando
    entry: W = -1;
  state Idle
    entry:W = 0;
  state Subiendo_hasta_arriba
    entry: W = 1;
  state Subiendo
    entry: W = 1;
  Subiendo -> Bajand_hasta_abajo [order 4] : [UI==4]
  Bajand_hasta_abajo -> Bajando [order 2] : [UI==3]
  Subiendo -> Bajando [order 3] : [UI==3]
  Bajando -> Bajand_hasta_abajo [order 2] : [UI==4]
  Idle -> Bajando [order 3] : [UI==3&&S>PosMinW4]
  Subiendo_hasta_arriba -> Bajand_hasta_abajo [order 3] : [UI==4]
  Idle -> Bajand_hasta_abajo [order 4] : [UI==4&&S>PosMinW4]
  Bajando -> Subiendo [order 3] : [UI==1]
  Subiendo_hasta_arriba -> Bajando [order 4] : [UI==3]
  Bajand_hasta_abajo -> Subiendo [order 4] : [UI==1]
  Bajand_hasta_abajo -> Idle [order 1] : [S<=PosMinW4]
  Bajand_hasta_abajo -> Subiendo_hasta_arriba [order 3] : [UI==2]
  Bajando -> Idle [order 1] : [S<=PosMinW4||UI==0]
  Bajando -> Subiendo_hasta_arriba [order 4] : [UI==2]
  (default) -> Idle
  Idle -> Subiendo_hasta_arriba [order 2] : [UI==2&&S<5]
  Idle -> Subiendo [order 1] : [UI == 1&&S<5]
  Subiendo -> Idle [order 1] : [S>=5||UI==0]
  Subiendo_hasta_arriba -> Idle [order 1] : [S >=5]
  Subiendo_hasta_arriba -> Subiendo [order 2] : [UI ==1]
  Subiendo -> Subiendo_hasta_arriba [order 2] : [UI==2]
  data: S input; UI input; W output double; PosMinW4 input

== stateflow chart c00003M_harness/M030/Cyber/WL/Chart ==
  state Bajand_hasta_abajo
    entry: W = -1;
  state Bajando
    entry: W = -1;
  state Idle
    entry:W = 0;
  state Subiendo_hasta_arriba
    entry: W = 1;
  state Subiendo
    entry: W = 1;
  Subiendo -> Bajand_hasta_abajo [order 4] : [UI==4]
  Bajand_hasta_abajo -> Bajando [order 2] : [UI==3]
  Subiendo -> Bajando [order 3] : [UI==3]
  Bajando -> Bajand_hasta_abajo [order 2] : [UI==4]
  Idle -> Bajando [order 3] : [UI==3&&S>0]
  Subiendo_hasta_arriba -> Bajand_hasta_abajo [order 3] : [UI==4]
  Idle -> Bajand_hasta_abajo [order 4] : [UI==4&&S>0]
  Bajando -> Subiendo [order 3] : [UI==1]
  Subiendo_hasta_arriba -> Bajando [order 4] : [UI==3]
  Bajand_hasta_abajo -> Subiendo [order 4] : [UI==1]
  Bajand_hasta_abajo -> Idle [order 1] : [S<=0]
  Bajand_hasta_abajo -> Subiendo_hasta_arriba [order 3] : [UI==2]
  Bajando -> Idle [order 1] : [S<=0||UI==0]
  Bajando -> Subiendo_hasta_arriba [order 4] : [UI==2]
  (default) -> Idle
  Idle -> Subiendo_hasta_arriba [order 2] : [UI==2&&S<5]
  Idle -> Subiendo [order 1] : [UI == 1&&S<5]
  Subiendo -> Idle [order 1] : [S>=5||UI==0]
  Subiendo_hasta_arriba -> Idle [order 1] : [S >=5]
  Subiendo_hasta_arriba -> Subiendo [order 2] : [UI ==1]
  Subiendo -> Subiendo_hasta_arriba [order 2] : [UI==2]
  data: S input; UI input; W output double

== stateflow chart c00003M_harness/M030/Cyber/WL1/Chart1 ==
  state Bajand_hasta_abajo
    entry: W = -1;
  state Bajando
    entry: W = -1;
  state Idle
    entry:W = 0;
  state Subiendo_hasta_arriba
    entry: W = 1;
  state Subiendo
    entry: W = 1;
  Subiendo -> Bajand_hasta_abajo [order 4] : [UI==4]
  Bajand_hasta_abajo -> Bajando [order 2] : [UI==3]
  Subiendo -> Bajando [order 3] : [UI==3]
  Bajando -> Bajand_hasta_abajo [order 2] : [UI==4]
  Idle -> Bajando [order 3] : [UI==3&&S>0]
  Subiendo_hasta_arriba -> Bajand_hasta_abajo [order 3] : [UI==4]
  Idle -> Bajand_hasta_abajo [order 4] : [UI==4&&S>0]
  Bajando -> Subiendo [order 3] : [UI==1]
  Subiendo_hasta_arriba -> Bajando [order 4] : [UI==3]
  Bajand_hasta_abajo -> Subiendo [order 4] : [UI==1]
  Bajand_hasta_abajo -> Idle [order 1] : [S<=0]
  Bajand_hasta_abajo -> Subiendo_hasta_arriba [order 3] : [UI==2]
  Bajando -> Idle [order 1] : [S<=0||UI==0]
  Bajando -> Subiendo_hasta_arriba [order 4] : [UI==2]
  (default) -> Idle
  Idle -> Subiendo_hasta_arriba [order 2] : [UI==2&&S<5]
  Idle -> Subiendo [order 1] : [UI == 1&&S<5]
  Subiendo -> Idle [order 1] : [S>=5||UI==0]
  Subiendo_hasta_arriba -> Idle [order 1] : [S >=5]
  Subiendo_hasta_arriba -> Subiendo [order 2] : [UI ==1]
  Subiendo -> Subiendo_hasta_arriba [order 2] : [UI==2]
  data: S input; UI input; W output double

== stateflow chart c00003M_harness/M030/Cyber/WL2/Chart1 ==
  state Bajand_hasta_abajo
    entry: W = -1;
  state Bajando
    entry: W = -1;
  state Idle
    entry:W = 0;
  state Subiendo_hasta_arriba
    entry: W = 1;
  state Subiendo
    entry: W = 1;
  Subiendo -> Bajand_hasta_abajo [order 4] : [UI==4]
  Bajand_hasta_abajo -> Bajando [order 2] : [UI==3]
  Subiendo -> Bajando [order 3] : [UI==3]
  Bajando -> Bajand_hasta_abajo [order 2] : [UI==4]
  Idle -> Bajando [order 3] : [UI==3&&S>PosMinW3]
  Subiendo_hasta_arriba -> Bajand_hasta_abajo [order 3] : [UI==4]
  Idle -> Bajand_hasta_abajo [order 4] : [UI==4&&S>PosMinW3]
  Bajando -> Subiendo [order 3] : [UI==1]
  Subiendo_hasta_arriba -> Bajando [order 4] : [UI==3]
  Bajand_hasta_abajo -> Subiendo [order 4] : [UI==1]
  Bajand_hasta_abajo -> Idle [order 1] : [S<=PosMinW3]
  Bajand_hasta_abajo -> Subiendo_hasta_arriba [order 3] : [UI==2]
  Bajando -> Idle [order 1] : [S<=PosMinW3||UI==0]
  Bajando -> Subiendo_hasta_arriba [order 4] : [UI==2]
  (default) -> Idle
  Idle -> Subiendo_hasta_arriba [order 2] : [UI==2&&S<5]
  Idle -> Subiendo [order 1] : [UI == 1&&S<5]
  Subiendo -> Idle [order 1] : [S>=5||UI==0]
  Subiendo_hasta_arriba -> Idle [order 1] : [S >=5]
  Subiendo_hasta_arriba -> Subiendo [order 2] : [UI ==1]
  Subiendo -> Subiendo_hasta_arriba [order 2] : [UI==2]
  data: S input; UI input; W output double; PosMinW3 input

== stateflow chart c00003M_harness/M030/Cyber/WL3/Chart2 ==
  state Bajand_hasta_abajo
    entry: W = -1;
  state Bajando
    entry: W = -1;
  state Idle
    entry:W = 0;
  state Subiendo_hasta_arriba
    entry: W = 1;
  state Subiendo
    entry: W = 0;
  Subiendo -> Bajand_hasta_abajo [order 4] : [UI==4]
  Bajand_hasta_abajo -> Bajando [order 2] : [UI==3]
  Subiendo -> Bajando [order 3] : [UI==3]
  Bajando -> Bajand_hasta_abajo [order 2] : [UI==4]
  Idle -> Bajando [order 3] : [UI==3&&S>PosMinW4]
  Subiendo_hasta_arriba -> Bajand_hasta_abajo [order 3] : [UI==4]
  Idle -> Bajand_hasta_abajo [order 4] : [UI==4&&S>PosMinW4]
  Bajando -> Subiendo [order 3] : [UI==1]
  Subiendo_hasta_arriba -> Bajando [order 4] : [UI==3]
  Bajand_hasta_abajo -> Subiendo [order 4] : [UI==1]
  Bajand_hasta_abajo -> Idle [order 1] : [S<=PosMinW4]
  Bajand_hasta_abajo -> Subiendo_hasta_arriba [order 3] : [UI==2]
  Bajando -> Idle [order 1] : [S<=PosMinW4||UI==0]
  Bajando -> Subiendo_hasta_arriba [order 4] : [UI==2]
  (default) -> Idle
  Idle -> Subiendo_hasta_arriba [order 2] : [UI==2&&S<5]
  Idle -> Subiendo [order 1] : [UI == 1&&S<5]
  Subiendo -> Idle [order 1] : [S>=5||UI==0]
  Subiendo_hasta_arriba -> Idle [order 1] : [S >=5]
  Subiendo_hasta_arriba -> Subiendo [order 2] : [UI ==1]
  Subiendo -> Subiendo_hasta_arriba [order 2] : [UI==2]
  data: S input; UI input; W output double; PosMinW4 input

== stateflow chart c00003M_harness/M031/Cyber/WL/Chart ==
  state Bajand_hasta_abajo
    entry: W = -1;
  state Bajando
    entry: W = -1;
  state Idle
    entry:W = 0;
  state Subiendo_hasta_arriba
    entry: W = 0;
  state Subiendo
    entry: W = 1;
  Subiendo -> Bajand_hasta_abajo [order 4] : [UI==4]
  Bajand_hasta_abajo -> Bajando [order 2] : [UI==3]
  Subiendo -> Bajando [order 3] : [UI==3]
  Bajando -> Bajand_hasta_abajo [order 2] : [UI==4]
  Idle -> Bajando [order 3] : [UI==3&&S>0]
  Subiendo_hasta_arriba -> Bajand_hasta_abajo [order 3] : [UI==4]
  Idle -> Bajand_hasta_abajo [order 4] : [UI==4&&S>0]
  Bajando -> Subiendo [order 3] : [UI==1]
  Subiendo_hasta_arriba -> Bajando [order 4] : [UI==3]
  Bajand_hasta_abajo -> Subiendo [order 4] : [UI==1]
  Bajand_hasta_abajo -> Idle [order 1] : [S<=0]
  Bajand_hasta_abajo -> Subiendo_hasta_arriba [order 3] : [UI==2]
  Bajando -> Idle [order 1] : [S<=0||UI==0]
  Bajando -> Subiendo_hasta_arriba [order 4] : [UI==2]
  (default) -> Idle
  Idle -> Subiendo_hasta_arriba [order 2] : [UI==2&&S<5]
  Idle -> Subiendo [order 1] : [UI == 1&&S<5]
  Subiendo -> Idle [order 1] : [S>=5||UI==0]
  Subiendo_hasta_arriba -> Idle [order 1] : [S >=5]
  Subiendo_hasta_arriba -> Subiendo [order 2] : [UI ==1]
  Subiendo -> Subiendo_hasta_arriba [order 2] : [UI==2]
  data: S input; UI input; W output double

== stateflow chart c00003M_harness/M031/Cyber/WL1/Chart1 ==
  state Bajand_hasta_abajo
    entry: W = -1;
  state Bajando
    entry: W = -1;
  state Idle
    entry:W = 0;
  state Subiendo_hasta_arriba
    entry: W = 1;
  state Subiendo
    entry: W = 1;
  Subiendo -> Bajand_hasta_abajo [order 4] : [UI==4]
  Bajand_hasta_abajo -> Bajando [order 2] : [UI==3]
  Subiendo -> Bajando [order 3] : [UI==3]
  Bajando -> Bajand_hasta_abajo [order 2] : [UI==4]
  Idle -> Bajando [order 3] : [UI==3&&S>0]
  Subiendo_hasta_arriba -> Bajand_hasta_abajo [order 3] : [UI==4]
  Idle -> Bajand_hasta_abajo [order 4] : [UI==4&&S>0]
  Bajando -> Subiendo [order 3] : [UI==1]
  Subiendo_hasta_arriba -> Bajando [order 4] : [UI==3]
  Bajand_hasta_abajo -> Subiendo [order 4] : [UI==1]
  Bajand_hasta_abajo -> Idle [order 1] : [S<=0]
  Bajand_hasta_abajo -> Subiendo_hasta_arriba [order 3] : [UI==2]
  Bajando -> Idle [order 1] : [S<=0||UI==0]
  Bajando -> Subiendo_hasta_arriba [order 4] : [UI==2]
  (default) -> Idle
  Idle -> Subiendo_hasta_arriba [order 2] : [UI==2&&S<5]
  Idle -> Subiendo [order 1] : [UI == 1&&S<5]
  Subiendo -> Idle [order 1] : [S>=5||UI==0]
  Subiendo_hasta_arriba -> Idle [order 1] : [S >=5]
  Subiendo_hasta_arriba -> Subiendo [order 2] : [UI ==1]
  Subiendo -> Subiendo_hasta_arriba [order 2] : [UI==2]
  data: S input; UI input; W output double

== stateflow chart c00003M_harness/M031/Cyber/WL2/Chart1 ==
  state Bajand_hasta_abajo
    entry: W = -1;
  state Bajando
    entry: W = -1;
  state Idle
    entry:W = 0;
  state Subiendo_hasta_arriba
    entry: W = 1;
  state Subiendo
    entry: W = 1;
  Subiendo -> Bajand_hasta_abajo [order 4] : [UI==4]
  Bajand_hasta_abajo -> Bajando [order 2] : [UI==3]
  Subiendo -> Bajando [order 3] : [UI==3]
  Bajando -> Bajand_hasta_abajo [order 2] : [UI==4]
  Idle -> Bajando [order 3] : [UI==3&&S>PosMinW3]
  Subiendo_hasta_arriba -> Bajand_hasta_abajo [order 3] : [UI==4]
  Idle -> Bajand_hasta_abajo [order 4] : [UI==4&&S>PosMinW3]
  Bajando -> Subiendo [order 3] : [UI==1]
  Subiendo_hasta_arriba -> Bajando [order 4] : [UI==3]
  Bajand_hasta_abajo -> Subiendo [order 4] : [UI==1]
  Bajand_hasta_abajo -> Idle [order 1] : [S<=PosMinW3]
  Bajand_hasta_abajo -> Subiendo_hasta_arriba [order 3] : [UI==2]
  Bajando -> Idle [order 1] : [S<=PosMinW3||UI==0]
  Bajando -> Subiendo_hasta_arriba [order 4] : [UI==2]
  (default) -> Idle
  Idle -> Subiendo_hasta_arriba [order 2] : [UI==2&&S<5]
  Idle -> Subiendo [order 1] : [UI == 1&&S<5]
  Subiendo -> Idle [order 1] : [S>=5||UI==0]
  Subiendo_hasta_arriba -> Idle [order 1] : [S >=5]
  Subiendo_hasta_arriba -> Subiendo [order 2] : [UI ==1]
  Subiendo -> Subiendo_hasta_arriba [order 2] : [UI==2]
  data: S input; UI input; W output double; PosMinW3 input

== stateflow chart c00003M_harness/M031/Cyber/WL3/Chart2 ==
  state Bajand_hasta_abajo
    entry: W = -1;
  state Bajando
    entry: W = -1;
  state Idle
    entry:W = 0;
  state Subiendo_hasta_arriba
    entry: W = 1;
  state Subiendo
    entry: W = 1;
  Subiendo -> Bajand_hasta_abajo [order 4] : [UI==4]
  Bajand_hasta_abajo -> Bajando [order 2] : [UI==3]
  Subiendo -> Bajando [order 3] : [UI==3]
  Bajando -> Bajand_hasta_abajo [order 2] : [UI==4]
  Idle -> Bajando [order 3] : [UI==3&&S>PosMinW4]
  Subiendo_hasta_arriba -> Bajand_hasta_abajo [order 3] : [UI==4]
  Idle -> Bajand_hasta_abajo [order 4] : [UI==4&&S>PosMinW4]
  Bajando -> Subiendo [order 3] : [UI==1]
  Subiendo_hasta_arriba -> Bajando [order 4] : [UI==3]
  Bajand_hasta_abajo -> Subiendo [order 4] : [UI==1]
  Bajand_hasta_abajo -> Idle [order 1] : [S<=PosMinW4]
  Bajand_hasta_abajo -> Subiendo_hasta_arriba [order 3] : [UI==2]
  Bajando -> Idle [order 1] : [S<=PosMinW4||UI==0]
  Bajando -> Subiendo_hasta_arriba [order 4] : [UI==2]
  (default) -> Idle
  Idle -> Subiendo_hasta_arriba [order 2] : [UI==2&&S<5]
  Idle -> Subiendo [order 1] : [UI == 1&&S<5]
  Subiendo -> Idle [order 1] : [S>=5||UI==0]
  Subiendo_hasta_arriba -> Idle [order 1] : [S >=5]
  Subiendo_hasta_arriba -> Subiendo [order 2] : [UI ==1]
  Subiendo -> Subiendo_hasta_arriba [order 2] : [UI==2]
  data: S input; UI input; W output double; PosMinW4 input

== stateflow chart c00003M_harness/M032/Cyber/WL/Chart ==
  state Bajand_hasta_abajo
    entry: W = -1;
  state Bajando
    entry: W = -1;
  state Idle
    entry:W = 0;
  state Subiendo_hasta_arriba
    entry: W = 1;
  state Subiendo
    entry: W = 1;
  Subiendo -> Bajand_hasta_abajo [order 4] : [UI==4]
  Bajand_hasta_abajo -> Bajando [order 2] : [UI==3]
  Subiendo -> Bajando [order 3] : [UI==3]
  Bajando -> Bajand_hasta_abajo [order 2] : [UI==4]
  Idle -> Bajando [order 3] : [UI==3&&S>0]
  Subiendo_hasta_arriba -> Bajand_hasta_abajo [order 3] : [UI==4]
  Idle -> Bajand_hasta_abajo [order 4] : [UI==4&&S>0]
  Bajando -> Subiendo [order 3] : [UI==1]
  Subiendo_hasta_arriba -> Bajando [order 4] : [UI==3]
  Bajand_hasta_abajo -> Subiendo [order 4] : [UI==1]
  Bajand_hasta_abajo -> Idle [order 1] : [S<=0]
  Bajand_hasta_abajo -> Subiendo_hasta_arriba [order 3] : [UI==2]
  Bajando -> Idle [order 1] : [S<=0||UI==0]
  Bajando -> Subiendo_hasta_arriba [order 4] : [UI==2]
  (default) -> Idle
  Idle -> Subiendo_hasta_arriba [order 2] : [UI==2&&S<5]
  Idle -> Subiendo [order 1] : [UI == 1&&S<5]
  Subiendo -> Idle [order 1] : [S>=5||UI==0]
  Subiendo_hasta_arriba -> Idle [order 1] : [S >=5]
  Subiendo_hasta_arriba -> Subiendo [order 2] : [UI ==1]
  Subiendo -> Subiendo_hasta_arriba [order 2] : [UI==2]
  data: S input; UI input; W output double

== stateflow chart c00003M_harness/M032/Cyber/WL1/Chart1 ==
  state Bajand_hasta_abajo
    entry: W = -1;
  state Bajando
    entry: W = -1;
  state Idle
    entry:W = 0;
  state Subiendo_hasta_arriba
    entry: W = 0;
  state Subiendo
    entry: W = 1;
  Subiendo -> Bajand_hasta_abajo [order 4] : [UI==4]
  Bajand_hasta_abajo -> Bajando [order 2] : [UI==3]
  Subiendo -> Bajando [order 3] : [UI==3]
  Bajando -> Bajand_hasta_abajo [order 2] : [UI==4]
  Idle -> Bajando [order 3] : [UI==3&&S>0]
  Subiendo_hasta_arriba -> Bajand_hasta_abajo [order 3] : [UI==4]
  Idle -> Bajand_hasta_abajo [order 4] : [UI==4&&S>0]
  Bajando -> Subiendo [order 3] : [UI==1]
  Subiendo_hasta_arriba -> Bajando [order 4] : [UI==3]
  Bajand_hasta_abajo -> Subiendo [order 4] : [UI==1]
  Bajand_hasta_abajo -> Idle [order 1] : [S<=0]
  Bajand_hasta_abajo -> Subiendo_hasta_arriba [order 3] : [UI==2]
  Bajando -> Idle [order 1] : [S<=0||UI==0]
  Bajando -> Subiendo_hasta_arriba [order 4] : [UI==2]
  (default) -> Idle
  Idle -> Subiendo_hasta_arriba [order 2] : [UI==2&&S<5]
  Idle -> Subiendo [order 1] : [UI == 1&&S<5]
  Subiendo -> Idle [order 1] : [S>=5||UI==0]
  Subiendo_hasta_arriba -> Idle [order 1] : [S >=5]
  Subiendo_hasta_arriba -> Subiendo [order 2] : [UI ==1]
  Subiendo -> Subiendo_hasta_arriba [order 2] : [UI==2]
  data: S input; UI input; W output double

== stateflow chart c00003M_harness/M032/Cyber/WL2/Chart1 ==
  state Bajand_hasta_abajo
    entry: W = -1;
  state Bajando
    entry: W = -1;
  state Idle
    entry:W = 0;
  state Subiendo_hasta_arriba
    entry: W = 1;
  state Subiendo
    entry: W = 1;
  Subiendo -> Bajand_hasta_abajo [order 4] : [UI==4]
  Bajand_hasta_abajo -> Bajando [order 2] : [UI==3]
  Subiendo -> Bajando [order 3] : [UI==3]
  Bajando -> Bajand_hasta_abajo [order 2] : [UI==4]
  Idle -> Bajando [order 3] : [UI==3&&S>PosMinW3]
  Subiendo_hasta_arriba -> Bajand_hasta_abajo [order 3] : [UI==4]
  Idle -> Bajand_hasta_abajo [order 4] : [UI==4&&S>PosMinW3]
  Bajando -> Subiendo [order 3] : [UI==1]
  Subiendo_hasta_arriba -> Bajando [order 4] : [UI==3]
  Bajand_hasta_abajo -> Subiendo [order 4] : [UI==1]
  Bajand_hasta_abajo -> Idle [order 1] : [S<=PosMinW3]
  Bajand_hasta_abajo -> Subiendo_hasta_arriba [order 3] : [UI==2]
  Bajando -> Idle [order 1] : [S<=PosMinW3||UI==0]
  Bajando -> Subiendo_hasta_arriba [order 4] : [UI==2]
  (default) -> Idle
  Idle -> Subiendo_hasta_arriba [order 2] : [UI==2&&S<5]
  Idle -> Subiendo [order 1] : [UI == 1&&S<5]
  Subiendo -> Idle [order 1] : [S>=5||UI==0]
  Subiendo_hasta_arriba -> Idle [order 1] : [S >=5]
  Subiendo_hasta_arriba -> Subiendo [order 2] : [UI ==1]
  Subiendo -> Subiendo_hasta_arriba [order 2] : [UI==2]
  data: S input; UI input; W output double; PosMinW3 input

== stateflow chart c00003M_harness/M032/Cyber/WL3/Chart2 ==
  state Bajand_hasta_abajo
    entry: W = -1;
  state Bajando
    entry: W = -1;
  state Idle
    entry:W = 0;
  state Subiendo_hasta_arriba
    entry: W = 1;
  state Subiendo
    entry: W = 1;
  Subiendo -> Bajand_hasta_abajo [order 4] : [UI==4]
  Bajand_hasta_abajo -> Bajando [order 2] : [UI==3]
  Subiendo -> Bajando [order 3] : [UI==3]
  Bajando -> Bajand_hasta_abajo [order 2] : [UI==4]
  Idle -> Bajando [order 3] : [UI==3&&S>PosMinW4]
  Subiendo_hasta_arriba -> Bajand_hasta_abajo [order 3] : [UI==4]
  Idle -> Bajand_hasta_abajo [order 4] : [UI==4&&S>PosMinW4]
  Bajando -> Subiendo [order 3] : [UI==1]
  Subiendo_hasta_arriba -> Bajando [order 4] : [UI==3]
  Bajand_hasta_abajo -> Subiendo [order 4] : [UI==1]
  Bajand_hasta_abajo -> Idle [order 1] : [S<=PosMinW4]
  Bajand_hasta_abajo -> Subiendo_hasta_arriba [order 3] : [UI==2]
  Bajando -> Idle [order 1] : [S<=PosMinW4||UI==0]
  Bajando -> Subiendo_hasta_arriba [order 4] : [UI==2]
  (default) -> Idle
  Idle -> Subiendo_hasta_arriba [order 2] : [UI==2&&S<5]
  Idle -> Subiendo [order 1] : [UI == 1&&S<5]
  Subiendo -> Idle [order 1] : [S>=5||UI==0]
  Subiendo_hasta_arriba -> Idle [order 1] : [S >=5]
  Subiendo_hasta_arriba -> Subiendo [order 2] : [UI ==1]
  Subiendo -> Subiendo_hasta_arriba [order 2] : [UI==2]
  data: S input; UI input; W output double; PosMinW4 input

== stateflow chart c00003M_harness/M033/Cyber/WL/Chart ==
  state Bajand_hasta_abajo
    entry: W = -1;
  state Bajando
    entry: W = -1;
  state Idle
    entry:W = 0;
  state Subiendo_hasta_arriba
    entry: W = 1;
  state Subiendo
    entry: W = 1;
  Subiendo -> Bajand_hasta_abajo [order 4] : [UI==4]
  Bajand_hasta_abajo -> Bajando [order 2] : [UI==3]
  Subiendo -> Bajando [order 3] : [UI==3]
  Bajando -> Bajand_hasta_abajo [order 2] : [UI==4]
  Idle -> Bajando [order 3] : [UI==3&&S>0]
  Subiendo_hasta_arriba -> Bajand_hasta_abajo [order 3] : [UI==4]
  Idle -> Bajand_hasta_abajo [order 4] : [UI==4&&S>0]
  Bajando -> Subiendo [order 3] : [UI==1]
  Subiendo_hasta_arriba -> Bajando [order 4] : [UI==3]
  Bajand_hasta_abajo -> Subiendo [order 4] : [UI==1]
  Bajand_hasta_abajo -> Idle [order 1] : [S<=0]
  Bajand_hasta_abajo -> Subiendo_hasta_arriba [order 3] : [UI==2]
  Bajando -> Idle [order 1] : [S<=0||UI==0]
  Bajando -> Subiendo_hasta_arriba [order 4] : [UI==2]
  (default) -> Idle
  Idle -> Subiendo_hasta_arriba [order 2] : [UI==2&&S<5]
  Idle -> Subiendo [order 1] : [UI == 1&&S<5]
  Subiendo -> Idle [order 1] : [S>=5||UI==0]
  Subiendo_hasta_arriba -> Idle [order 1] : [S >=5]
  Subiendo_hasta_arriba -> Subiendo [order 2] : [UI ==1]
  Subiendo -> Subiendo_hasta_arriba [order 2] : [UI==2]
  data: S input; UI input; W output double

== stateflow chart c00003M_harness/M033/Cyber/WL1/Chart1 ==
  state Bajand_hasta_abajo
    entry: W = -1;
  state Bajando
    entry: W = -1;
  state Idle
    entry:W = 0;
  state Subiendo_hasta_arriba
    entry: W = 1;
  state Subiendo
    entry: W = 1;
  Subiendo -> Bajand_hasta_abajo [order 4] : [UI==4]
  Bajand_hasta_abajo -> Bajando [order 2] : [UI==3]
  Subiendo -> Bajando [order 3] : [UI==3]
  Bajando -> Bajand_hasta_abajo [order 2] : [UI==4]
  Idle -> Bajando [order 3] : [UI==3&&S>0]
  Subiendo_hasta_arriba -> Bajand_hasta_abajo [order 3] : [UI==4]
  Idle -> Bajand_hasta_abajo [order 4] : [UI==4&&S>0]
  Bajando -> Subiendo [order 3] : [UI==1]
  Subiendo_hasta_arriba -> Bajando [order 4] : [UI==3]
  Bajand_hasta_abajo -> Subiendo [order 4] : [UI==1]
  Bajand_hasta_abajo -> Idle [order 1] : [S<=0]
  Bajand_hasta_abajo -> Subiendo_hasta_arriba [order 3] : [UI==2]
  Bajando -> Idle [order 1] : [S<=0||UI==0]
  Bajando -> Subiendo_hasta_arriba [order 4] : [UI==2]
  (default) -> Idle
  Idle -> Subiendo_hasta_arriba [order 2] : [UI==2&&S<5]
  Idle -> Subiendo [order 1] : [UI == 1&&S<5]
  Subiendo -> Idle [order 1] : [S>=5||UI==0]
  Subiendo_hasta_arriba -> Idle [order 1] : [S >=5]
  Subiendo_hasta_arriba -> Subiendo [order 2] : [UI ==1]
  Subiendo -> Subiendo_hasta_arriba [order 2] : [UI==2]
  data: S input; UI input; W output double

== stateflow chart c00003M_harness/M033/Cyber/WL2/Chart1 ==
  state Bajand_hasta_abajo
    entry: W = -1;
  state Bajando
    entry: W = -1;
  state Idle
    entry:W = 0;
  state Subiendo_hasta_arriba
    entry: W = 0;
  state Subiendo
    entry: W = 1;
  Subiendo -> Bajand_hasta_abajo [order 4] : [UI==4]
  Bajand_hasta_abajo -> Bajando [order 2] : [UI==3]
  Subiendo -> Bajando [order 3] : [UI==3]
  Bajando -> Bajand_hasta_abajo [order 2] : [UI==4]
  Idle -> Bajando [order 3] : [UI==3&&S>PosMinW3]
  Subiendo_hasta_arriba -> Bajand_hasta_abajo [order 3] : [UI==4]
  Idle -> Bajand_hasta_abajo [order 4] : [UI==4&&S>PosMinW3]
  Bajando -> Subiendo [order 3] : [UI==1]
  Subiendo_hasta_arriba -> Bajando [order 4] : [UI==3]
  Bajand_hasta_abajo -> Subiendo [order 4] : [UI==1]
  Bajand_hasta_abajo -> Idle [order 1] : [S<=PosMinW3]
  Bajand_hasta_abajo -> Subiendo_hasta_arriba [order 3] : [UI==2]
  Bajando -> Idle [order 1] : [S<=PosMinW3||UI==0]
  Bajando -> Subiendo_hasta_arriba [order 4] : [UI==2]
  (default) -> Idle
  Idle -> Subiendo_hasta_arriba [order 2] : [UI==2&&S<5]
  Idle -> Subiendo [order 1] : [UI == 1&&S<5]
  Subiendo -> Idle [order 1] : [S>=5||UI==0]
  Subiendo_hasta_arriba -> Idle [order 1] : [S >=5]
  Subiendo_hasta_arriba -> Subiendo [order 2] : [UI ==1]
  Subiendo -> Subiendo_hasta_arriba [order 2] : [UI==2]
  data: S input; UI input; W output double; PosMinW3 input
